simulink library "mci_models"  (R2020a)
settings: Solver=VariableStepAuto  StartTime=0.0  StopTime=10.0  RelTol=1e-3
undefined symbols (not defined in the file): x0
(part 1 of 2)
Description:
  | Library of MCI specific blocks and models.
  | 
  | Release 2023
settings Model: Creator=Andreas Mehrle  LastModifiedBy=User
settings DataIOCC: ReturnWorkspaceOutputs=off
settings DebuggingCC: ArithmeticOperatorsInVariantConditions=warning
settings SFSimCC: SimUseLocalCustomCode=off  CustomCodeUndefinedFunction=UseInterfaceOnly
settings RTWCC: RTWUseLocalCustomCode=off
settings CodeAppCC: StateflowObjectComments=on

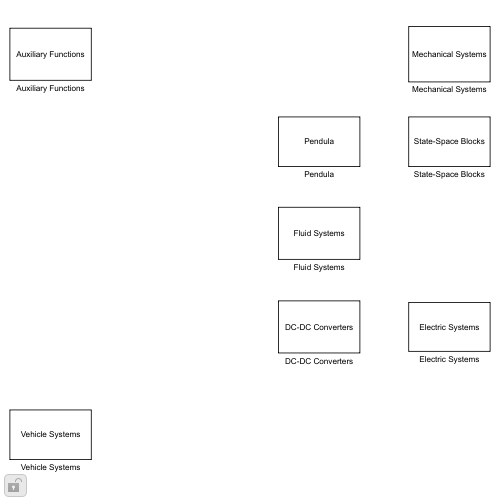
[thumbnail: Simulink's stored preview of the top-level diagram]
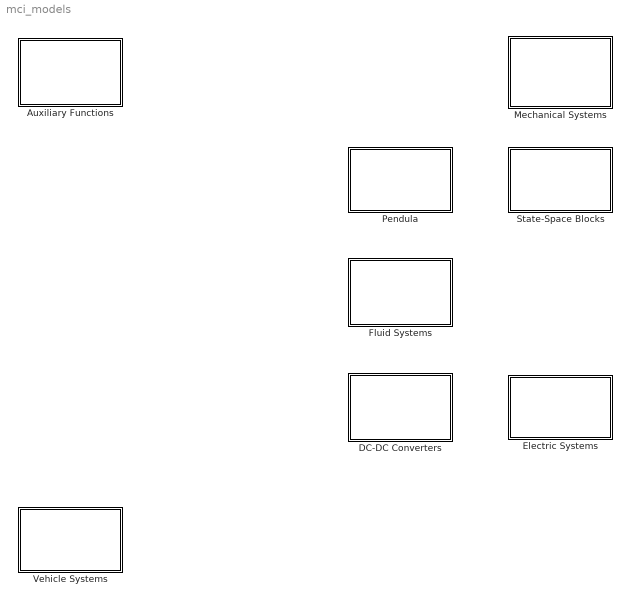
== system mci_models ==
  Auxiliary Functions : Subsystem
      mask Display: disp(get_param(gcb,'Name'))
  DC-DC Converters : Subsystem
      mask Display: disp(get_param(gcb,'Name'))
  Electric Systems : Subsystem
      mask Display: disp(get_param(gcb,'Name'))
  Fluid Systems : Subsystem
      mask Display: disp(get_param(gcb,'Name'))
  Mechanical Systems : Subsystem
      mask Display: disp(get_param(gcb,'Name'))
  Pendula : Subsystem
      mask Display: disp(get_param(gcb,'Name'))
  State-Space Blocks : Subsystem
      mask Display: disp(get_param(gcb,'Name'))
  Vehicle Systems : Subsystem
      mask Display: disp(get_param(gcb,'Name'))

== system mci_models/Auxiliary Functions ==
  Friction model : Subsystem  mask(Friction Function){c=[1 20 0.5 0]}
      mask prompts: c "Friction parameters"
      mask help:
      | Block computes non-linear friction coefficient.
      |
      | Inputs:
      |  - v ... vehicle velocity (m/s)
      |  - v_w ... wheel velocity (m/s)
      |
      | Outputs:
      |  - lambda ... slip
      |  - mu ... friction coefficient
      mask init:
      | p.c=c;
      mask DialogControl DescTextVar Prompt: Engine characteristics
      mask Display:
      | l=0:1/20:1;
      | m=c(1)*(1-exp(-c(2)*l))-c(3)*l;
      | 
      | color('white')
      | plot([-0.2 -0.2],[-0.2 1.3]);
      | plot([-0.2 1.3],[-0.2 -0.2]);
      | 
      | color('black')
      | plot(l,m)
      | plot([0 1 1 0 0],[0 0 1 1 0])
      | %plot([0 0],[0 1])
      | %text(1.1,0.09,'l')
      | %text(0.02,1.2,'mu')
      | 
      | port_label('input',1,'v')
      | port_label('input',2,'v_w','texmode','on')
      | port_label('output',1,'\lambda','texmode','on')
      | port_label('output',2,'\mu','texmode','on')
  Polynomial : Subsystem  mask(Polynomial Function){p=[-4 4 0]}
      mask prompts: p "Coefficients ([p_n p_n-1 ... p_1 p_0])"
      mask help: Establishes polynomial relation between input and output.
      mask DialogControl DescTextVar Prompt: Engine characteristics
      mask Display:
      | wmax=max(roots(p));
      | w=0:wmax/10:wmax;
      | %wmax=max(w);
      | ymax=max(polyval(p,w));
      | 
      | color('white')
      | plot([-0.2*wmax -0.2*wmax],[-0.2*ymax 1.3*ymax]);
      | plot([-0.2*wmax 1.3*wmax],[-0.2*ymax -0.2*ymax]);
      | 
      | color('black')
      | plot(w,polyval(p,w))
      | plot([0 wmax wmax 0 0],[0 0 ymax ymax 0])
      | %plot([0 0],[0 ymax])
      | %text(1.1*wmax,0.09*ymax,'u')
      | %text(0.02*wmax,1.2*ymax,'y')
      | 
      | %port_label('input',1,'u')
      | %port_label('output',1,'y')
  Trajectory : Subsystem  mask(Trajectory Generator){t1=1, dt=1, y1=0, y2=1, n=5, m=0}
      mask prompts: t1 "Start time (s)"; dt "Duration (s)"; y1 "Start value"; y2 "End value"; n "Order"; m "Derivatives"
      mask help:
      | Generates polynomial trajectory of different order with smooth beginning and end.
      |
      | Inputs: none
      |
      | Outputs:
      |  - y ... trajectory
      |  - dy ... time derivative of y (optional)
      |  - ddy ... second derivative of y (optional)
      |
      | Before start time and after ending y is kept constant and all derivatives become 0.
      mask init:
      | p.t1=t1;
      |     p.t2=t1+dt;
      |     p.dt=dt;
      |     p.y1=y1;
      |     p.y2=y2;
      | 
      |     p.n=str2num(get_param(gcb,'n'));
      |     if p.n==3
      |         p.p=[-2 3 0 0];
      |         p.dp=[-6 6 0];
      |         p.ddp=[-12 6];
      |     elseif p.n==5
      |         p.p=[6 -15 10 0 0 0];
      |         p.dp=[30 -60 30 0 0];
      |         p.ddp=[120 -180 60 0];
      |     elseif p.n==7
      |         p.p=[-20 70 -84 35 0 0 0 0];
      |         p.dp=[-140 420 -420 140 0 0 0];
      |         p.ddp=[-840 2100 -1680 420 0 0];
      |     end
      | 
      |     p.m=str2num(get_param(gcb,'m'));
      |     if p.m==0
      |         if (getSimulinkBlockHandle([gcb, '/dy']) ~= -1)             % If it DOES exist (dy)
      |                 ho = get_param([gcb, '/dy'], 'LineHandles');        % we get the line handles to eliminate them first
      |                 delete_line(ho.Inport);                             % we delete the line
      |                 delete_block([gcb, '/dy']);                    % we delete the block
      |         end
      |         if (getSimulinkBlockHandle([gcb, '/ddy']) ~= -1)             % If it DOES exist (dy)
      |                 ho = get_param([gcb, '/ddy'], 'LineHandles');        % we get the line handles to eliminate them first
      |                 delete_line(ho.Inport);                             % we delete the line
      |                 delete_block([gcb, '/ddy']);                    % we delete the block
      |         end
      |     elseif p.m==1
      |         if (getSimulinkBlockHandle([gcb, '/dy']) == -1)             % If it DOES NOT exist (dy)
      |                 add_block('simulink/Sinks/Out1',[gcb, '/dy']);% add the block
      |                 set_param([gcb, '/dy'],'position',[285    53   315    67]);    % we place it somewhere
      |                 ho = get_param([gcb, '/dy'], 'PortHandles');               % we get the port handles of the new inport port
      |                 gen = get_param([gcb, '/tragen'], 'PortHandles');           % we get the port handles of the product block
      |                 add_line(gcb,gen.Outport(2),ho.Inport(1));                       % we create the connection between new input outport and appropriate product inport
      |         end
      |         if (getSimulinkBlockHandle([gcb, '/ddy']) ~= -1)             % If it DOES exist (dy)
      |                 ho = get_param([gcb, '/ddy'], 'LineHandles');        % we get the line handles to eliminate them first
      |                 delete_line(ho.Inport);                             % we delete the line
      |                 delete_block([gcb, '/ddy']);                    % we delete the block
      |         end
      |     elseif p.m==2
      |         if (getSimulinkBlockHandle([gcb, '/dy']) == -1)             % If it DOES NOT exist (dy)
      |                 add_block('simulink/Sinks/Out1',[gcb, '/dy']);% add the block
      |                 set_param([gcb, '/dy'],'position',[285    53   315    67]);    % we place it somewhere
      |                 ho = get_param([gcb, '/dy'], 'PortHandles');               % we get the port handles of the new inport port
      |                 gen = get_param([gcb, '/tragen'], 'PortHandles');           % we get the port handles of the product block
      |                 add_line(gcb,gen.Outport(2),ho.Inport(1));                       % we create the connection between new input outport and appropriate product inport
      |         end
      |         if (getSimulinkBlockHandle([gcb, '/ddy']) == -1)             % If it DOES NOT exist (dy)
      |                 add_block('simulink/Sinks/Out1',[gcb, '/ddy']);% add the block
      |                 set_param([gcb, '/ddy'],'position',[285    88   315   102]);    % we place it somewhere
      |                 ho = get_param([gcb, '/ddy'], 'PortHandles');               % we get the port handles of the new inport port
      |                 gen = get_param([gcb, '/tragen'], 'PortHandles');           % we get the port handles of the product block
      |                 add_line(gcb,gen.Outport(3),ho.Inport(1));                       % we create the connection between new input outport and appropriate product inport
      |         end
      | 
      |     end
      mask TypeOptions n: 3 | 5 | 7
      mask TypeOptions m: 0 | 1 | 2
      mask DialogControl DescTextVar Prompt: Engine characteristics
      mask Display:
      | t=0:p.dt/10:p.dt;
      | tmax=p.t2;
      | y=p.y1+(p.y2-p.y1)*polyval(p.p,t/p.dt);
      | ymax=max(y);
      | 
      | color('white')
      | plot([-0.2*tmax -0.2*tmax],[-0.2*ymax 1.3*ymax]);
      | plot([-0.2*tmax 1.3*tmax],[-0.2*ymax -0.2*ymax]);
      | 
      | color('black')
      | plot([0 t+p.t1],[p.y1 y])
      | plot([0 tmax tmax 0 0],[0 0 ymax ymax 0])
      | %plot([0 0],[0 ymax])
      | %text(1.1*tmax,0.09*ymax,'t')
      | %text(0.02*tmax,1.2*ymax,'y')
      | text(0.1*tmax,0.8*ymax,['n=',num2str(p.n)])
      | 
      | %port_label('output',1,'y')
      | %if p.n>1
      | %    port_label('output',2,'\dot{y}','texmode','on')
      | %end

== system mci_models/DC-DC Converters ==
  Buck Converter : Subsystem  mask{L=1, R=1, C=1, G=1, ui=1, x0=[0;0]}
      mask prompts: L "L (H)"; R "R (Ohm)"; C "C (F)"; G "G (S)"; ui "Supply voltage (V)"; x0 "Initial state [i_L;u_C]"
      mask DialogControl DescTextVar Prompt: Cuk Converter
      mask Display:
      | % labels
      | %port_label('input',1,'u_i','texmode','on')
      | %port_label('input',2,'d')
      | %port_label('output',1,'x')
      | % circuit
      | plot([0.15 0.30],[0.7 0.7])
      | plot([0.29 0.4 0.85 0.85],[0.6 0.7 0.7 0.6])
      | %patch([0.15 0.3 0.3 0.15 0.15],[0.73 0.73 0.62 0.62 0.73],[0 0 0])
      | %plot([0.39 0.39],[0.8 0.6])
      | %plot([0.415 0.415],[0.8 0.6])
      | patch([0.47 0.62 0.62 0.47 0.47],[0.73 0.73 0.62 0.62 0.73],[0 0 0])
      | %plot([0.35 0.35 0.4],[0.7 0.5 0.5])
      | %plot([0.45 0.45],[0.7 0.5])
      | plot([0.3 0.3],[0.62 0.2])
      | plot([0.7 0.7],[0.7 0.47])
      | plot([0.65 0.75],[0.47 0.47])
      | plot([0.65 0.75],[0.43 0.43])
      | plot([0.7 0.7],[0.43 0.2])
      | plot([0.815 0.875 0.875 0.815 0.815],[0.6 0.6 0.3 0.3 0.6])
      | plot([0.15 0.85 0.85],[0.2 0.2 0.3])
  Cuk Converter : Subsystem  mask{L1=1, R1=1, C1=1, L2=1, R2=1, C2=1, G=1, ui=1, x0_copy=[0;0;1e-6;0]}
      mask prompts: L1 "L1 (H)"; R1 "R1 (Ohm)"; C1 "C1 (F)"; L2 "L2 (H)"; R2 "R2 (Ohm)"; C2 "C2 (F)"; G "G (S)"; ui "Supply voltage"; x0_copy "Initial state [i1;i2;uc1;uc2]"
      mask init:
      | p.L1=L1;
      | p.R1=R1;
      | p.C1=C1;
      | p.L2=L2;
      | p.R2=R2;
      | p.C2=C2;
      | p.G=G;
      | p.ui=ui;
      mask DialogControl DescTextVar Prompt: Cuk Converter
      mask Display:
      | % labels
      | %port_label('input',1,'u_i','texmode','on')
      | %port_label('input',2,'d')
      | %port_label('output',1,'x')
      | % circuit
      | plot([0.05 0.39],[0.7 0.7])
      | plot([0.415 0.9 0.9],[0.7 0.7 0.6])
      | patch([0.15 0.3 0.3 0.15 0.15],[0.73 0.73 0.62 0.62 0.73],[0 0 0])
      | plot([0.39 0.39],[0.8 0.6])
      | plot([0.415 0.415],[0.8 0.6])
      | patch([0.5 0.65 0.65 0.5 0.5],[0.73 0.73 0.62 0.62 0.73],[0 0 0])
      | plot([0.35 0.35 0.4],[0.7 0.5 0.5])
      | plot([0.45 0.45],[0.7 0.5])
      | plot([0.38 0.45 0.45],[0.53 0.35 0.2])
      | plot([0.75 0.75],[0.7 0.47])
      | plot([0.7 0.8],[0.47 0.47])
      | plot([0.7 0.8],[0.43 0.43])
      | plot([0.75 0.75],[0.43 0.2])
      | plot([0.865 0.925 0.925 0.865 0.865],[0.6 0.6 0.3 0.3 0.6])
      | plot([0.1 0.9 0.9],[0.2 0.2 0.3])
  RL-Load : Subsystem  mask{L=1, R=1, ui=1, x0=0}
      mask prompts: L "L (H)"; R "R (Ohm)"; ui "Supply voltage (V)"; x0 "Initial state [i_L]"
      mask DialogControl DescTextVar Prompt: Cuk Converter
      mask Display:
      | % labels
      | %port_label('input',1,'u_i','texmode','on')
      | %port_label('input',1,'d')
      | %port_label('output',1,'x')
      | % circuit
      | plot([0.15 0.50 0.5 0.55],[0.9 0.9 0.8 0.7])
      | plot([0.3 0.3 0.35],[0.9 0.8 0.7])
      | plot([0.3 0.3 0.35],[0.7 0.3 0.2])
      | plot([0.3 0.3],[0.2 0.1])
      | plot([0.5 0.5 0.55],[0.7 0.3 0.2])
      | plot([0.5 0.8 0.8 0.3],[0.6 0.6 0.4 0.4])
      | patch([0.65 0.75 0.75 0.65],[0.375 0.375 0.425 0.425],[0 0 0])
      | %plot([0.3 0.3],[0.62 0.2])
      | %plot([0.7 0.7],[0.7 0.47])
      | %plot([0.65 0.75],[0.47 0.47])
      | %plot([0.65 0.75],[0.43 0.43])
      | %plot([0.7 0.7],[0.43 0.2])
      | %plot([0.815 0.875 0.875 0.815 0.815],[0.6 0.6 0.3 0.3 0.6])
      | plot([0.15 0.5 0.5],[0.1 0.1 0.2])

== system mci_models/Electric Systems ==
  GPS-IMU Sensor : Subsystem  mask{T=1, D=1, var_IMU=0.1, a0=0.1}
      mask prompts: T "Sampling time (s)"; D "Quantization (m)"; var_IMU "Noise variation (m^2/s^4)"; a0 "Offset (m/s^2)"
      mask DialogControl Container3 Prompt: GPS
      mask DialogControl Container4 Prompt: IMU
      mask Display:
      | image(imread('grafics/gyro.png'))
      | 
      | % labels
      | port_label('input',1,'u')
      | port_label('output',1,'y_{GPS}','texmode','on')
      | port_label('output',2,'a_{IMU}','texmode','on')
  Magnetic Levitation : Subsystem  mask{y0=1, m=1, R=1, L0=1, L1=1, g=9.81, x0=[0;0;0]}
      mask prompts: y0 "Operating distance (m)"; m "Levitated mass (kg)"; R "Coil resistance (Ohm)"; L0 "Coil inductance (H)"; L1 "Sphere inductance (H)"; g "Gravitational acceleration (m/s^2)"; x0 "Initial state [y;v;i]"
      mask init:
      | p.y0=y0;
      | p.m=m;
      | p.R=R;
      | p.L0=L0;
      | p.L1=L1;
      | p.g=g;
      mask Display:
      | patch([0.580 0.576 0.565 0.547 0.525 0.500 0.475 0.453 0.435 0.424 0.420 0.424 0.435 0.453 0.475 0.500 0.525 0.547 0.565 0.576 0.580 ],[0.500 0.533 0.563 0.586 0.601 0.607 0.601 0.586 0.563 0.533 0.500 0.467 0.437 0.414 0.399 0.393 0.399 0.414 0.437 0.467 0.500 ])
      | patch([0.4 0.6 0.6 0.4],[0.95 0.95 0.85 0.85],[0.5 0.5 0.5])
      | plot([0.177 0.250 0.330 0.414 0.500 0.586 0.670 0.750 0.823 ],[0.407 0.347 0.303 0.276 0.267 0.276 0.303 0.347 0.407 ])
      | plot([0.235 0.296 0.361 0.430 0.500 0.570 0.639 0.704 0.765 ],[0.515 0.465 0.429 0.407 0.400 0.407 0.429 0.465 0.515 ])
      | plot([0.294 0.341 0.392 0.445 0.500 0.555 0.608 0.659 0.706 ],[0.622 0.584 0.556 0.539 0.533 0.539 0.556 0.584 0.622 ])
      | plot([0.353 0.387 0.423 0.461 0.500 0.539 0.577 0.613 0.647 ],[0.730 0.703 0.683 0.671 0.667 0.671 0.683 0.703 0.730 ])
      | plot([0.7 0.1 0.1 0.6],[0 0 1 1])
      | % labels
      | port_label('input',1,'u')
      | port_label('output',1,'x')

== system mci_models/Fluid Systems ==
  Bioreactor : Subsystem  mask{cg0=0, mu0=0, k0=0, k1=0, k2=0, alpha=0, x0=[0;0]}
      mask prompts: cg0 "Inflow concentration glucose (kg/m^3)"; mu0 "Growth rate (1/[t])"; k0 "Affinity constant (kg/m^3)"; k1 "Linear affinity constant"; k2 "Quadratic affinity constant (m^3/kg)"; alpha "Yield rate"; x0 "Initial state [c_c;c_g]"
      mask init:
      | p.cg0=cg0;
      | p.mu0=mu0;
      | p.k0=k0;
      | p.k1=k1;
      | p.k2=k2;
      | p.alpha=alpha;
      mask Display:
      | image(imread('grafics/bioreactor.png'))
      | 
      | port_label('input',1,'q')
      | port_label('output',1,'c')
  Fan Model : Subsystem  mask{K1=1, tau1=1, K2=1, tau2=1, w_on=1, w_off=1, sensorType=off, T=1}
      mask prompts: K1 "Gain (rad/s V)"; tau1 "Time constant (s)"; K2 "Gain (rad/s V)"; tau2 "Time constant (s)"; w_on "Breakoff speed (rad/s)"; w_off "Freeze speed (rad/s)"; sensorType "Enable discrete sensing"; T "Sampling time for discrete sensing (s)"
      mask init:
      | p.T=T;
      | maskHandle=Simulink.Mask.get(gcb);
      | if sensorType==1
      |     set_param([gcb,'/Sensor1'],'Commented','off');
      |     set_param([gcb,'/Sensor2'],'Commented','off');
      |     maskHandle.Parameters(1,8).Enabled='on';
      | else
      |     set_param([gcb,'/Sensor1'],'Commented','through');
      |     set_param([gcb,'/Sensor2'],'Commented','through');
      |     maskHandle.Parameters(1,8).Enabled='off';
      | end
      mask DialogControl DescTextVar Prompt: BB8 model
      mask DialogControl Fan1 Prompt: Fan 1
      mask DialogControl Fan2 Prompt: Fan 2
      mask DialogControl Container5 Prompt: Sensor
      mask Display:
      | image(imread('grafics/turbine.png'))
      | 
      | port_label('input',1,'u')
      | port_label('output',1,'w1')
      | port_label('output',2,'w2')
  Pneumatic Cylinder : Subsystem  mask{m=1, A=1, k=1, b=0.1, x0=[1;0]}
      mask prompts: m "Piston mass (kg)"; A "Piston area (m^2)"; k "Spring konstant (N/m)"; b "Friction constant (N s/m)"; x0 "Initial state [x;v] (p will be chosen to match the spring force)"
      mask init:
      | p.m=m;
      | p.A=A;
      | p.k=k;
      | p.b=b;
      | x0(3)=x0(1)*p.k/p.A;
      mask DialogControl DescTextVar Prompt: Nonlinear pneumatic cylinder with ideal gas properties.
      mask Display:
      | % bar
      | plot([0.35,0.9],[0.5,0.5])
      | % piston
      | %plot([0.4,0.4,0.35,0.35,0.4],[0.3,0.7,0.7,0.3,0.3])
      | patch([0.42,0.42,0.38,0.38,0.42],[0.3,0.66,0.66,0.3,0.3],[0.5,0.5,0.5])
      | % case
      | plot([0.65,0.65,0.1,0.1,0.65,0.65],[0.475,0.3,0.3,0.7,0.7,0.525])
      | % spring
      | plot([0.4,0.45,0.5,0.55,0.6,0.65],[0.3,0.7,0.3,0.7,0.3,0.7])
      | % labels
      | port_label('input',1,'q')
      | port_label('output',1,'x')
  Tank with Outflow : Subsystem  mask{At=1, Ao=0.1, rho=1, zeta=0, g=9.81, h0=1}
      mask prompts: At "Tank section (m^2)"; Ao "Outflow section (m^2)"; rho "Fluid density (kg/m^3)"; zeta "Friction loss coefficient"; g "Gravitational acceleration (m/s^2)"; h0 "Initial height (m)"
      mask init:
      | p.At=At;
      | p.Ao=Ao;
      | p.rho=rho;
      | p.zeta=zeta;
      | p.g=g;
      mask DialogControl DescTextVar Prompt: Nonlinear tank with outflow
      mask Display:
      | patch([0.35 0.35 0.3 0.3],[0.75 0.6 0.6 0.75],[0.5 0.5 0.5])
      | patch([0.25 0.75 0.75 0.25],[0.6 0.6 0.2 0.2],[0.5 0.5 0.5])
      | patch([0.47 0.53 0.53 0.47],[0.2 0.2 0.05 0.05],[0.5 0.5 0.5])
      | plot([0.1 0.34 0.34 0.27 0.27 0.1],[1 1 0.8 0.8 0.88 0.88])
      | plot([0.22 0.22 0.44 0.44],[0.7 0.18 0.18 0.12])
      | plot([0.76 0.76 0.53 0.53],[0.7 0.18 0.18 0.12])
      | 
      | port_label('input',1,'qi')
      | port_label('output',1,'h')
      | port_label('output',2,'qo')

== system mci_models/Mechanical Systems ==
  Elevator : Subsystem  mask{m=1, J=1, r=1, g=9.81, b1=1, b2=0.1, k=1e3, x0=[0;1;0;0], display=off}
      mask prompts: m "Mass cabin (kg)"; J "Moment of inertia engine (kg m^2)"; r "Wheel radius (m)"; g "Gravitational acceleration (m/s^2)"; b1 "Translational friction (N s/m)"; b2 "Rotational friction (N m s)"; k "Rope stiffness (N)"; x0 "Initial state [x;phi;v;w]"; display "Activate real-time visualization"
      mask init:
      | p.r=r;
      | p.m=m;
      | p.J=J;
      | p.g=g;
      | p.b1=b1;
      | p.b2=b2;
      | p.k=k;
      | %x0(2)=x0(1)/(r*(m*g/k+1));
      settings: MinAlgLoopOccurrences=on
      mask DialogControl DescTextVar Prompt: Nonlinear pendulum on cart model
      mask Display:
      | plot([0,1],[0.05,0.05])
      | plot([0.4,0.4,0.6,0.6,0.4],[0.2,0.5,0.5,0.2,0.2])
      | plot([0.5,0.5],[0.5,1])
      | % labels
      | port_label('input',1,'M')
      | port_label('output',1,'x')
      | port_label('output',2,'e')
  Lunar Lander : Subsystem  mask{vt=0, g=9.81, x0=[1;0;1]}
      mask prompts: vt "Thruster exit velocity (m/s)"; g "Gravitational acceleration (m/s^2)"; x0 "Initial state [h,v,m]"
      mask init:
      | p.vt=vt;
      | p.g=g;
      mask DialogControl DescTextVar Prompt: Lunar Lander Model
      mask Display:
      | image(imread('grafics/lander.png'))
      | 
      | port_label('input',1,'q')
      | port_label('output',1,'x')
  Segway Model : Subsystem  mask{m0=1, m1=1, I0=0, I1=0, r=1, s=1, b0=1, b1=0, g=9.81, x0=[0;0;0;0], display=on}
      mask prompts: m0 "Wheel mass (kg)"; m1 "Pendulum mass (kg)"; I0 "Wheel moment of inertia (kg m^2)"; I1 "Pendulum moment of inertia (kg m^2)"; r "Wheel radius"; s "Distance of pendulum COG from hub (m)"; b0 "Rolling friction coefficient wheel (N m s/rad)"; b1 "Turning friction coefficient hub (N m s/rad)"; g "Gravitational acceleration (m/s^2)"; x0 "Initial state [a;w;da;dw]"; display "Activate real-time visualization"
      mask init:
      | p.m0=m0;
      | p.m1=m1;
      | p.I0=(m0+m1)*r^2+I0;
      | p.I1=m1*s^2+I1;
      | p.I01=m1*r*s;
      | p.b1=b1;
      | if b1==0;
      |     p.nu=b0/1e-6;
      | else
      |     p.nu=b0/b1;
      | end
      | p.g=g/r;
      mask DialogControl DescTextVar Prompt: BB8 model
      mask Display:
      | image(imread('grafics/segway.png'))
      | 
      | port_label('input',1,'M')
      | port_label('output',1,'x')

== system mci_models/Pendula ==
  Double Pendulum on Cart : Subsystem  mask{s1=1, s2=1, l1=1, m0=1, m1=1, m2=1, I1=0, I2=0, g=9.81, b0=0.1, b1=0.1, b2=0.1, x0=[0;0;0;0;0;0], display=off}
      mask prompts: s1 "Distance of pendulum 1 COG from hinge point (m)"; s2 "Distance of pendulum 2 COG from hinge point (m)"; l1 "Length of pendulum 1 (m)"; m0 "Mass cart (kg)"; m1 "Mass pendulum 1 (kg)"; m2 "Mass pendulum 2 (kg)"; I1 "Moment of inertia pendulum 1 (kg m^2)"; I2 "Moment of inertia pendulum 2 (kg m^2)"; g "Gravitational acceleration (m/s^2)"; b0 "Translational friction (N s/m)"; b1 "Rotational friction joint 1 (N m s)"; b2 "Rotational friction joint 2 (N m s)"; x0 "Initial state [x;phi1;phi2;v;w1;w2]"; display "Activate real-time visualization"
      mask init:
      | p.M=m0+m1+m2;
      | p.I11=I1+m1*s1^2+m2*l1^2;
      | p.I22=I2+m2*s2^2;
      | p.I12=m2*l1*s2;
      | p.I2p=m2*s2;
      | p.I12p=m1*s1+m2*l1;
      | p.g=g;
      | p.b0=b0;
      | p.b1=b1;
      | p.b2=b2;
      mask Display:
      | plot([0,1],[0.05,0.05])
      | plot([0.3,0.3,0.7,0.7,0.3],[0.1,0.4,0.4,0.1,0.1])
      | plot([0.5,0.6,0.4],[0.25,0.65,1])
      | % labels
      | port_label('input',1,'F')
      | port_label('output',1,'x')
  Mathematical Pendulum : Subsystem  mask{m=1, l=1, k=0, b=0.1, g=9.81, x0=[0;0], display=off}
      mask prompts: m "Mass (kg)"; l "Pendulum length (m)"; k "Spring constant (N m/rad)"; b "Friction coefficient (N m s/rad)"; g "Gravitational acceleration (m/s^2)"; x0 "Initial state [phi;w]"; display "Activate real-time visualization"
      mask init:
      | p.m=m;
      | p.l=l;
      | p.k=k;
      | p.b=b;
      | p.g=g;
      mask DialogControl DescTextVar Prompt: Nonlinear mathematical pendulum
      mask Display:
      | % support
      | plot([0.3 0.7],[1 1])
      | plot([0.45 0.5 0.55],[1 0.9 1])
      | % pendulum
      | plot([0.5 0.33],[0.9 0.22])
      | text(0.3,0.2,'O')
      | % labels
      | port_label('input',1,'M')
      | port_label('output',1,'x')
  Motion Controlled Double Pendulum : Subsystem  mask{g=9.81, x0=[0;0;0;0;0], display=off, l1=1, m2=1, m1=1, s2=1, s1=1, I2=0, b2=0.1, I1=0, b1=0.1}
      mask prompts: g "Gravitational acceleration (m/s^2)"; x0 "Initial state [x;phi1;phi2;w1;w2]"; display "Activate real-time visualization"; l1 "Length (m)"; m2 "Mass (kg)"; m1 "Mass (kg)"; s2 "Distance of COG from hinge point (m)"; s1 "Distance of COG from hinge point (m)"; I2 "Moment of inertia (kg m^2)"; b2 "Rotational friction (N m s)"; I1 "Moment of inertia (kg m^2)"; b1 "Rotational friction (N m s)"
      mask init:
      | p.I11=I1+m1*s1^2+m2*l1^2;
      | p.I22=I2+m2*s2^2;
      | p.I12=m2*l1*s2;
      | p.I2p=m2*s2;
      | p.I12p=m1*s1+m2*l1;
      | p.g=g;
      | p.b1=b1;
      | p.b2=b2;
      mask DialogControl Container3 Prompt: Pendulum 1
      mask DialogControl Container4 Prompt: Pendulum 2
      mask Display:
      | % ground
      | plot([0,1],[0.05,0.05])
      | % cart
      | plot([0.3,0.3,0.7,0.7,0.3],[0.1,0.3,0.3,0.1,0.1])
      | % pendulum
      | plot([0.5,0.6,0.4],[0.3,0.63,0.95])
      | % motion control
      | plot([0,0.3],[0.2,0.2])
      | plot([0.25,0.3,0.25],[0.15,0.2,0.25])
      | % labels
      | port_label('input',1,'v')
      | port_label('output',1,'x')
      | 
      | 
      | %plot([0,1],[0.05,0.05])
      | %plot([0.3,0.3,0.7,0.7,0.3],[0.1,0.4,0.4,0.1,0.1])
      | %plot([0.5,0.6,0.4],[0.25,0.65,1])
      | %plot([0,0.3],[0.25,0.25])
      | %plot([0.25,0.3,0.25],[0.2,0.25,0.3])
  Motion Controlled Pendulum : Subsystem  mask{s=1, m1=1, J=0, g=9.81, b1=0.1, x0=[0;0;0;0], display=off}
      mask prompts: s "Distance of pendulum COG from hinge point (m)"; m1 "Mass pendulum (kg)"; J "Moment of inertia pendulum"; g "Gravitational acceleration (m/s^2)"; b1 "Rotational friction (N m s)"; x0 "Initial state [x;phi;w]"; display "Activate real-time visualization"
      mask init:
      | p.s=s;
      | p.m1=m1;
      | p.J1=J;
      | p.g=g;
      | p.b1=b1;
      settings: MinAlgLoopOccurrences=on
      mask DialogControl DescTextVar Prompt: Nonlinear pendulum on cart model
      mask Display:
      | % ground
      | plot([0,1],[0.05,0.05])
      | % cart
      | plot([0.3,0.3,0.7,0.7,0.3],[0.1,0.3,0.3,0.1,0.1])
      | % pendulum
      | plot([0.5,0.6],[0.3,0.95])
      | % motion control
      | plot([0,0.3],[0.2,0.2])
      | plot([0.25,0.3,0.25],[0.15,0.2,0.25])
      | % labels
      | port_label('input',1,'v')
      | port_label('output',1,'x')
  Pendulum on Cart : Subsystem  Description=|  mask{s=1, m0=1, m1=1, J=0, g=9.81, b0=0, b1=0.1, x0=[0;0;0;0], display=off}
      | Simple model for pendulum on force driven slider. The states are x=[y v] where y is the
      | (horizontal) position and v the velocity of the slider. As input a force is taken u=F.
      | 
      | For the slider only its mass and the friction koefficient with the surface needs to be provided.
      | For the pendulum parameters include mass, distance of COG from hinge point, moment of
      | inertia around the COG for the pendulum and the friction coefficient of the rotatory motion.
      mask prompts: s "Distance of pendulum COG from hinge point (m)"; m0 "Mass cart (kg)"; m1 "Mass pendulum (kg)"; J "Moment of inertia pendulum"; g "Gravitational acceleration (m/s^2)"; b0 "Translational friction (N s/m)"; b1 "Rotational friction (N m s)"; x0 "Initial state [y;phi;v;w]"; display "Activate real-time visualization"
      mask init:
      | p.s=s;
      | p.m0=m0
      | p.m1=m1;
      | p.J=J;
      | p.g=g;
      | p.b0=b0;
      | p.b1=b1;
      settings: MinAlgLoopOccurrences=on
      mask DialogControl DescTextVar Prompt: Nonlinear pendulum on cart model
      mask Display:
      | plot([0,1],[0.05,0.05])
      | plot([0.3,0.3,0.7,0.7,0.3],[0.1,0.4,0.4,0.1,0.1])
      | plot([0.5,0.6],[0.25,1])
      | % labels
      | port_label('input',1,'F')
      | port_label('output',1,'x')

== system mci_models/State-Space Blocks ==
  Continuous State-Space : Subsystem  mask{A=1, B=1, C=1, D=1, x0=0}
      mask prompts: x0 "Initial conditions:"
      mask DialogControl DescTextVar Prompt: State-space model
      mask Display:
      | % annotation
      | text(0.5,0.6,'x''=Ax+Bu','horizontalAlignment','center')
      | text(0.5,0.4,'y=Cx+Du','horizontalAlignment','center')
      | % ports
      | port_label('input',1,'u')
      | port_label('output',1,'y')
      | port_label('output',2,'x')
  Discrete State-Space : Subsystem  mask{A=1, B=1, C=1, D=1, x0=0, T=1}
      mask prompts: x0 "Initial conditions:"; T "Sampling time"
      mask DialogControl DescTextVar Prompt: State-space model
      mask Display:
      | % annotation
      | text(0.5,0.6,texlabel('x_{k+1}=Ax_k+Bu_k'),'horizontalAlignment','center','Interpreter','tex')
      | text(0.5,0.4,'y_k=Cx_k+Du_k','horizontalAlignment','center','Interpreter','tex')
      | % ports
      | port_label('input',1,'u_k','Interpreter','tex')
      | port_label('output',1,'y_k','Interpreter','tex')
      | port_label('output',2,'x_k','Interpreter','tex')

== system mci_models/Vehicle Systems ==
  Car Dynamics : Subsystem  mask(Car Dynamics Model){m=1, cf=1, cd=1, rho=1.25, A=1, g=9.81, x0=0}
      mask prompts: m "Car mass (kg)"; cf "Friction coefficient"; cd "Drag coefficient"; rho "Air density (kg/m^3)"; A "Projected section area (m^2)"; g "Gravitational acceleration (m/s^2)"; x0 "Initial velocity [v0]"
      mask help:
      | Calculates the one-dimensional dynamics of a vehicle.
      |
      | Inputs:
      |  - phi ... road inclination (rad)
      |  - F ... thrust force (N)
      |
      | Outputs:
      |  - a ... acceleration (m/s^2)
      |  - v ... velocity (m/s)
      |
      | Mechanical (velocity proportional) and aerodynamic drag are considered by the respective coefficients.
      mask init:
      | p.m=m;
      | p.cd=cd;
      | p.cf=cf;
      | p.rho=rho;
      | p.A=A;
      | p.g=g;
      mask DialogControl DescTextVar Prompt: Car dynamics
      mask Display:
      | image(imread('grafics/car1.png'))
      | 
      | port_label('input',1,'\phi','texmode','on')
      | port_label('input',2,'F')
      | port_label('output',1,'a')
      | port_label('output',2,'v')
  Car Kinematics : Subsystem  mask(Car Kinematics Model){l=1, phimax=1, x0=[0;0;0]}
      mask prompts: l "Wheelbase (m)"; phimax "Maximum steering angle (rad)"; x0 "Initial state [x;y;phi]"
      mask help:
      | Computes two-dimensional (in-plane) kinematics of a vehicle.
      |
      | Inputs:
      |  - v ... translational velocity (m/s)
      |  - alpha ... steering angle (rad)
      |
      | Outputs:
      |  - x ... state [x-position, y-position, heading angle]
      |  - dx ... derivative of x [x-velocity, y-velocity, angular rotation rate]
      |
      | Steering angle can be limited to a maximum value.
      mask DialogControl DescTextVar Prompt: Kinematic model of a car
      mask Display:
      | image(imread('grafics/car2.png'))
      | 
      | port_label('input',1,'v')
      | port_label('input',2,'\alpha','texmode','on')
      | port_label('output',1,'x')
      | port_label('output',2,'dx')
      | % draw car
      | %patch([0.2 0.3 0.3 0.2],[0.73 0.73 0.7 0.7],[0 0 0])
      | %patch([0.7 0.8 0.8 0.7],[0.73 0.73 0.7 0.7],[0 0 0])
      | %plot([0.1 0.9 0.9 0.1 0.1],[0.7 0.7 0.3 0.3 0.7])
  Wheel Dynamics : Subsystem  mask(Wheel Dynamics Model){J=1, r=1, w0=0}
      mask prompts: J "Wheel moment of inertia (kg m^2)"; r "Radius (m)"; w0 "Initial velocity [w0]"
      mask help:
      | Computes wheel velocity from applied torque and road friction force. Usually used together with friction model.
      |
      | Inputs:
      |  - M ... engine torque (Nm)
      |  - F ... road friction force (N)
      |
      | Output:
      |  - v_w ... wheel velocity (m/s)
      |
      | Takes into account wheel dynamics by its moment of inertia.
      mask init:
      | p.J=J;
      | p.r=r;
      mask DialogControl DescTextVar Prompt: Car dynamics
      mask Display:
      | image(imread('grafics/wheel.png'))
      | 
      | port_label('input',1,'M')
      | port_label('input',2,'F')
      | port_label('output',1,'v_w','texmode','on')

== system mci_models/Auxiliary Functions/Friction model ==
  v : Inport
  w : Inport  Port=2
  MATLAB Function : MATLAB Function  TreatAsAtomicUnit=on
  l : Outport  VectorParamsAs1DForOutWhenUnconnected=off
  mu : Outport  Port=2  VectorParamsAs1DForOutWhenUnconnected=off
  wires:
  v/1 -> MATLAB Function/1(v)
  w/1 -> MATLAB Function/2(w)
  MATLAB Function/2(m) -> mu/1
  MATLAB Function/1(l) -> l/1

== system mci_models/Auxiliary Functions/Polynomial ==
  u : Inport
  MATLAB Function1 : MATLAB Function  TreatAsAtomicUnit=on
  y : Outport  VectorParamsAs1DForOutWhenUnconnected=off
  wires:
  MATLAB Function1/1(y) -> y/1
  u/1 -> MATLAB Function1/1(u)

== system mci_models/Auxiliary Functions/Trajectory ==
  Clock : Clock
  tragen : MATLAB Function  TreatAsAtomicUnit=on
  y : Outport  VectorParamsAs1DForOutWhenUnconnected=off
  wires:
  Clock/1 -> tragen/1(t)
  tragen/1(y) -> y/1

== system mci_models/DC-DC Converters/Buck Converter ==
  d : Inport
  Gain : Gain  Gain=[ui/L;0]  Multiplication=Matrix(K*u)
  Gain1 : Gain  Gain=[-R/L -1/L;1/C -G/C]  Multiplication=Matrix(K*u)
  Integrator : Integrator  InitialCondition=x0
  Sum : Sum  Inputs=|++
  x : Outport  VectorParamsAs1DForOutWhenUnconnected=off
  wires:
  Integrator/1 -> Gain1/1, x/1
  d/1 -> Gain/1
  Gain/1 -> Sum/1
  Sum/1 -> Integrator/1
  Gain1/1 -> Sum/2

== system mci_models/DC-DC Converters/Cuk Converter ==
  d : Inport
  Cuk converter1 : MATLAB Function  TreatAsAtomicUnit=on
  Integrator : Integrator  InitialCondition=x0
  x : Outport  VectorParamsAs1DForOutWhenUnconnected=off
  wires:
  d/1 -> Cuk converter1/1(d)
  Cuk converter1/1(dx) -> Integrator/1
  Integrator/1 -> x/1, Cuk converter1/2(x)

== system mci_models/DC-DC Converters/RL-Load ==
  d : Inport
  Gain : Gain  Gain=ui/L
  Gain1 : Gain  Gain=-R/L
  Integrator : Integrator  InitialCondition=x0
  Sum : Sum  Inputs=|++
  u : Outport  VectorParamsAs1DForOutWhenUnconnected=off
  wires:
  d/1 -> Gain/1
  Gain/1 -> Sum/1
  Sum/1 -> Integrator/1
  Integrator/1 -> Gain1/1, u/1
  Gain1/1 -> Sum/2

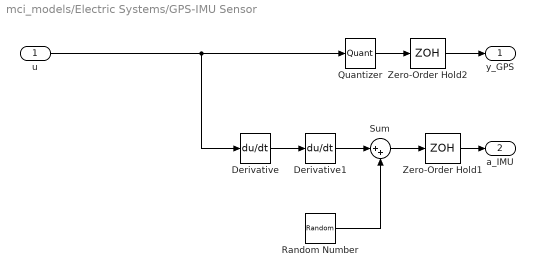
== system mci_models/Electric Systems/GPS-IMU Sensor ==
  u : Inport
  Derivative : Derivative
  Derivative1 : Derivative
  Quantizer : Quantizer  QuantizationInterval=D
  Random Number : RandomNumber  Mean=a0  Variance=var_IMU  Seed=rand()  SampleTime=T
  Sum : Sum  Inputs=|++
  Zero-Order Hold1 : ZeroOrderHold  SampleTime=T
  Zero-Order Hold2 : ZeroOrderHold  SampleTime=T
  y_GPS : Outport  VectorParamsAs1DForOutWhenUnconnected=off
  a_IMU : Outport  Port=2  VectorParamsAs1DForOutWhenUnconnected=off
  wires:
  Derivative/1 -> Derivative1/1
  Derivative1/1 -> Sum/1
  Random Number/1 -> Sum/2
  u/1 -> Derivative/1, Quantizer/1
  Quantizer/1 -> Zero-Order Hold2/1
  Zero-Order Hold2/1 -> y_GPS/1
  Zero-Order Hold1/1 -> a_IMU/1
  Sum/1 -> Zero-Order Hold1/1

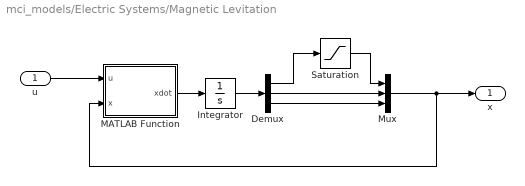
== system mci_models/Electric Systems/Magnetic Levitation ==
  u : Inport
  Demux : Demux  Outputs=3
  Integrator : Integrator  InitialCondition=x0
  MATLAB Function : MATLAB Function  TreatAsAtomicUnit=on
  Mux : Mux  Inputs=3
  Saturation : Saturate  UpperLimit=2*p.y0  LowerLimit=0
  x : Outport  VectorParamsAs1DForOutWhenUnconnected=off
  wires:
  u/1 -> MATLAB Function/1(u)
  MATLAB Function/1(xdot) -> Integrator/1
  Integrator/1 -> Demux/1
  Demux/1 -> Saturation/1
  Saturation/1 -> Mux/1
  Mux/1 -> MATLAB Function/2(x), x/1
  Demux/2 -> Mux/2
  Demux/3 -> Mux/3

== system mci_models/Fluid Systems/Bioreactor ==
  u : Inport
  Integrator : Integrator  InitialCondition=x0
  MATLAB Function : MATLAB Function  TreatAsAtomicUnit=on
  x : Outport  VectorParamsAs1DForOutWhenUnconnected=off
  wires:
  Integrator/1 -> MATLAB Function/2(x), x/1
  u/1 -> MATLAB Function/1(u)
  MATLAB Function/1(xdot) -> Integrator/1

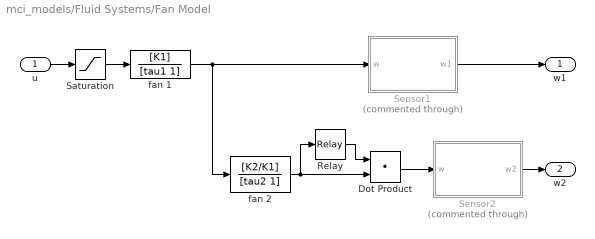
== system mci_models/Fluid Systems/Fan Model ==
  u : Inport
  Dot Product : DotProduct  InputSameDT=on  OutDataTypeStr=Inherit: Inherit via internal rule
  Relay : Relay  OnSwitchValue=w_on  OffSwitchValue=w_off
  Saturation : Saturate  UpperLimit=inf  LowerLimit=0
  Sensor1 : Subsystem  Commented=through
  Sensor2 : Subsystem  Commented=through
  fan 1 : TransferFcn  Numerator=[K1]  Denominator=[tau1 1]
  fan 2 : TransferFcn  Numerator=[K2/K1]  Denominator=[tau2 1]
  w1 : Outport  VectorParamsAs1DForOutWhenUnconnected=off
  w2 : Outport  Port=2  VectorParamsAs1DForOutWhenUnconnected=off
  wires:
  fan 1/1 -> fan 2/1, Sensor1/1(w)
  fan 2/1 -> Dot Product/2, Relay/1
  Relay/1 -> Dot Product/1
  Sensor1/1(w1) -> w1/1
  Dot Product/1 -> Sensor2/1(w)
  Sensor2/1(w2) -> w2/1
  Saturation/1 -> fan 1/1
  u/1 -> Saturation/1

== system mci_models/Fluid Systems/Pneumatic Cylinder ==
  p : Inport
  Integrator : Integrator  InitialCondition=x0
  MATLAB Function : MATLAB Function  TreatAsAtomicUnit=on
  x : Outport  VectorParamsAs1DForOutWhenUnconnected=off
  wires:
  Integrator/1 -> x/1, MATLAB Function/2(x)
  MATLAB Function/1(dx) -> Integrator/1
  p/1 -> MATLAB Function/1(u)

== system mci_models/Fluid Systems/Tank with Outflow ==
  q : Inport
  Integrator : Integrator  InitialCondition=h0
  MATLAB Function : MATLAB Function  TreatAsAtomicUnit=on
  h : Outport  VectorParamsAs1DForOutWhenUnconnected=off
  qo : Outport  Port=2  VectorParamsAs1DForOutWhenUnconnected=off
  wires:
  MATLAB Function/1(qo) -> qo/1
  MATLAB Function/2(hdot) -> Integrator/1
  Integrator/1 -> MATLAB Function/2(h), h/1
  q/1 -> MATLAB Function/1(qi)

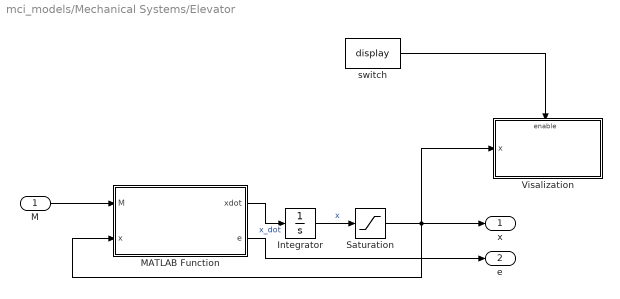
== system mci_models/Mechanical Systems/Elevator ==
  M : Inport
  Integrator : Integrator  InitialCondition=x0
  MATLAB Function : MATLAB Function  TreatAsAtomicUnit=on
  Saturation : Saturate  UpperLimit=[inf;inf;inf;inf]  LowerLimit=[-inf;1;-inf;-inf]
  Visalization : Subsystem  TreatAsAtomicUnit=on
  switch : Constant  Value=display
  x : Outport  VectorParamsAs1DForOutWhenUnconnected=off
  e : Outport  Port=2  VectorParamsAs1DForOutWhenUnconnected=off
  wires:
  M/1 -> MATLAB Function/1(M)
  Integrator/1 -> Saturation/1  "x"
  MATLAB Function/1(xdot) -> Integrator/1  "x_dot"
  switch/1 -> Visalization/Enable
  Saturation/1 -> Visalization/1(x), x/1, MATLAB Function/2(x)
  MATLAB Function/2(e) -> e/1

== system mci_models/Mechanical Systems/Lunar Lander ==
  q : Inport
  Integrator : Integrator  InitialCondition=x0
  MATLAB Function : MATLAB Function  TreatAsAtomicUnit=on
  Saturation : Saturate  UpperLimit=inf  LowerLimit=0
  x : Outport  VectorParamsAs1DForOutWhenUnconnected=off
  wires:
  MATLAB Function/1(xdot) -> Integrator/1
  Integrator/1 -> x/1, MATLAB Function/2(x)
  Saturation/1 -> MATLAB Function/1(u)
  q/1 -> Saturation/1

== system mci_models/Mechanical Systems/Segway Model ==
  M : Inport
  Integrator : Integrator  InitialCondition=x0
  MATLAB Function : MATLAB Function  TreatAsAtomicUnit=on
  display segway : Subsystem
  switch : Constant  Value=display
  x : Outport  VectorParamsAs1DForOutWhenUnconnected=off
  wires:
  switch/1 -> display segway/Enable
  MATLAB Function/1(dx) -> Integrator/1
  Integrator/1 -> MATLAB Function/2(x), x/1, display segway/1(x)
  M/1 -> MATLAB Function/1(u)

== system mci_models/Pendula/Double Pendulum on Cart ==
  F : Inport
  Enabled Subsystem : Subsystem  TreatAsAtomicUnit=on
  Integrator : Integrator  InitialCondition=x0
  MATLAB Function : MATLAB Function  TreatAsAtomicUnit=on
  switch : Constant  Value=display
  x : Outport  VectorParamsAs1DForOutWhenUnconnected=off
  wires:
  switch/1 -> Enabled Subsystem/Enable
  F/1 -> MATLAB Function/1(u), Enabled Subsystem/2(F)
  Integrator/1 -> MATLAB Function/2(x), x/1, Enabled Subsystem/1(x)
  MATLAB Function/1(xdot) -> Integrator/1

== system mci_models/Pendula/Mathematical Pendulum ==
  M : Inport
  Integrator : Integrator  InitialCondition=x0
  MATLAB Function : MATLAB Function  TreatAsAtomicUnit=on
  Visualization : Subsystem
  switch : Constant  Value=display
  x : Outport  VectorParamsAs1DForOutWhenUnconnected=off
  wires:
  MATLAB Function/1(xdot) -> Integrator/1
  M/1 -> MATLAB Function/1(u)
  Integrator/1 -> Visualization/1(x), MATLAB Function/2(x), x/1
  switch/1 -> Visualization/Enable

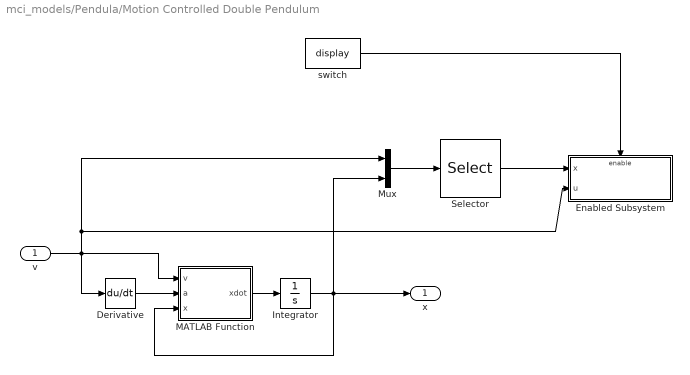
== system mci_models/Pendula/Motion Controlled Double Pendulum ==
  v : Inport
  Derivative : Derivative
  Enabled Subsystem : Subsystem  TreatAsAtomicUnit=on
  Integrator : Integrator  InitialCondition=x0
  MATLAB Function : MATLAB Function  TreatAsAtomicUnit=on
  Mux : Mux  Inputs=2
  Selector : Selector  InputPortWidth=6  IndexOptions=Index vector (dialog)  Indices=[2 3 4 1 5 6]  OutputSizes=1
  switch : Constant  Value=display
  x : Outport  VectorParamsAs1DForOutWhenUnconnected=off
  wires:
  switch/1 -> Enabled Subsystem/Enable
  v/1 -> Derivative/1, MATLAB Function/1(v), Mux/1, Enabled Subsystem/2(u)
  Integrator/1 -> Mux/2, MATLAB Function/3(x), x/1
  MATLAB Function/1(xdot) -> Integrator/1
  Derivative/1 -> MATLAB Function/2(a)
  Mux/1 -> Selector/1
  Selector/1 -> Enabled Subsystem/1(x)

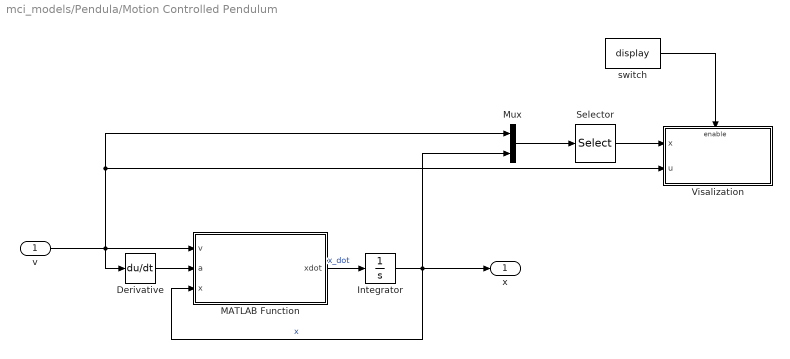
== system mci_models/Pendula/Motion Controlled Pendulum ==
  v : Inport
  Derivative : Derivative
  Integrator : Integrator  InitialCondition=x0
  MATLAB Function : MATLAB Function  TreatAsAtomicUnit=on
  Mux : Mux  Inputs=2
  Selector : Selector  InputPortWidth=4  IndexOptions=Index vector (dialog)  Indices=[2 3 1 4]  OutputSizes=1
  Visalization : Subsystem  TreatAsAtomicUnit=on
  switch : Constant  Value=display
  x : Outport  VectorParamsAs1DForOutWhenUnconnected=off
  wires:
  v/1 -> Visalization/2(u), Mux/1, Derivative/1, MATLAB Function/1(v)
  Integrator/1 -> Mux/2, x/1, MATLAB Function/3(x)  "x"
  MATLAB Function/1(xdot) -> Integrator/1  "x_dot"
  switch/1 -> Visalization/Enable
  Derivative/1 -> MATLAB Function/2(a)
  Mux/1 -> Selector/1
  Selector/1 -> Visalization/1(x)

== system mci_models/Pendula/Pendulum on Cart ==
  F : Inport
  Integrator : Integrator  InitialCondition=x0
  MATLAB Function : MATLAB Function  TreatAsAtomicUnit=on
  Visalization : Subsystem  TreatAsAtomicUnit=on
  switch : Constant  Value=display
  x : Outport  VectorParamsAs1DForOutWhenUnconnected=off
  wires:
  F/1 -> Visalization/2(u), MATLAB Function/1(F)
  Integrator/1 -> Visalization/1(x), x/1, MATLAB Function/2(x)  "x"
  MATLAB Function/1(xdot) -> Integrator/1  "x_dot"
  switch/1 -> Visalization/Enable

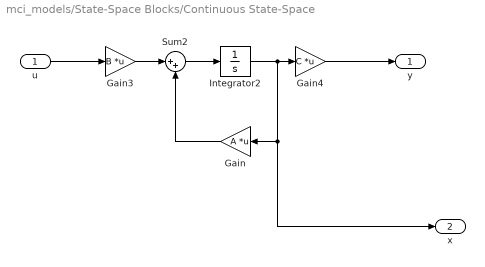
== system mci_models/State-Space Blocks/Continuous State-Space ==
  u : Inport
  Gain : Gain  Gain=A  Multiplication=Matrix(K*u)
  Gain3 : Gain  Gain=B  Multiplication=Matrix(K*u)
  Gain4 : Gain  Gain=C  Multiplication=Matrix(K*u)
  Integrator2 : Integrator  InitialCondition=x0
  Sum2 : Sum  Inputs=|++
  y : Outport  VectorParamsAs1DForOutWhenUnconnected=off
  x : Outport  Port=2  VectorParamsAs1DForOutWhenUnconnected=off
  wires:
  Integrator2/1 -> Gain4/1, Gain/1, x/1
  Gain3/1 -> Sum2/1
  Gain/1 -> Sum2/2
  Sum2/1 -> Integrator2/1
  Gain4/1 -> y/1
  u/1 -> Gain3/1

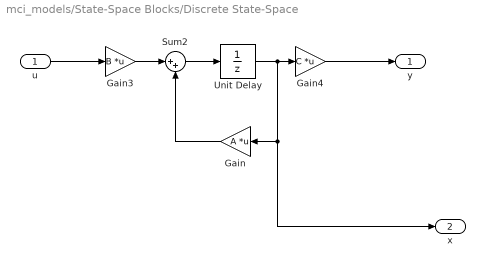
== system mci_models/State-Space Blocks/Discrete State-Space ==
  u : Inport
  Gain : Gain  Gain=A  Multiplication=Matrix(K*u)
  Gain3 : Gain  Gain=B  Multiplication=Matrix(K*u)
  Gain4 : Gain  Gain=C  Multiplication=Matrix(K*u)
  Sum2 : Sum  Inputs=|++
  Unit Delay : UnitDelay  InitialCondition=x0  SampleTime=T  HasFrameUpgradeWarning=on
  y : Outport  VectorParamsAs1DForOutWhenUnconnected=off
  x : Outport  Port=2  VectorParamsAs1DForOutWhenUnconnected=off
  wires:
  Unit Delay/1 -> Gain4/1, Gain/1, x/1
  Gain3/1 -> Sum2/1
  Gain/1 -> Sum2/2
  Sum2/1 -> Unit Delay/1
  Gain4/1 -> y/1
  u/1 -> Gain3/1

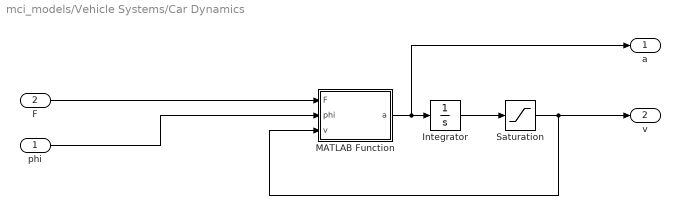
== system mci_models/Vehicle Systems/Car Dynamics ==
  phi : Inport
  F : Inport  Port=2
  Integrator : Integrator  InitialCondition=x0
  MATLAB Function : MATLAB Function  TreatAsAtomicUnit=on
  Saturation : Saturate  UpperLimit=inf  LowerLimit=0
  a : Outport  VectorParamsAs1DForOutWhenUnconnected=off
  v : Outport  Port=2  VectorParamsAs1DForOutWhenUnconnected=off
  wires:
  phi/1 -> MATLAB Function/2(phi)
  MATLAB Function/1(a) -> a/1, Integrator/1
  Integrator/1 -> Saturation/1
  F/1 -> MATLAB Function/1(F)
  Saturation/1 -> v/1, MATLAB Function/3(v)

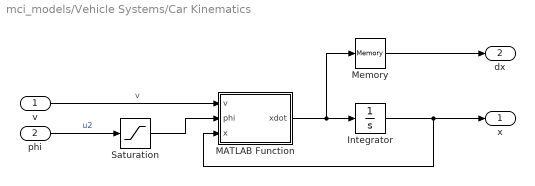
== system mci_models/Vehicle Systems/Car Kinematics ==
  v : Inport
  phi : Inport  Port=2
  Integrator : Integrator  InitialCondition=x0
  MATLAB Function : MATLAB Function  TreatAsAtomicUnit=on
  Memory : Memory
  Saturation : Saturate  UpperLimit=phimax  LowerLimit=-phimax
  x : Outport  VectorParamsAs1DForOutWhenUnconnected=off
  dx : Outport  Port=2  VectorParamsAs1DForOutWhenUnconnected=off
  wires:
  Integrator/1 -> MATLAB Function/3(x), x/1
  phi/1 -> Saturation/1  "u2"
  v/1 -> MATLAB Function/1(v)  "v"
  MATLAB Function/1(xdot) -> Memory/1, Integrator/1
  Memory/1 -> dx/1
  Saturation/1 -> MATLAB Function/2(phi)

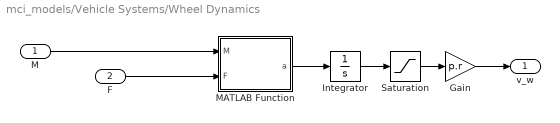
== system mci_models/Vehicle Systems/Wheel Dynamics ==
  M : Inport
  F : Inport  Port=2
  Gain : Gain  Gain=p.r
  Integrator : Integrator  InitialCondition=w0
  MATLAB Function : MATLAB Function  TreatAsAtomicUnit=on
  Saturation : Saturate  UpperLimit=inf  LowerLimit=0
  v_w : Outport  VectorParamsAs1DForOutWhenUnconnected=off
  wires:
  M/1 -> MATLAB Function/1(M)
  MATLAB Function/1(a) -> Integrator/1
  F/1 -> MATLAB Function/2(F)
  Gain/1 -> v_w/1
  Integrator/1 -> Saturation/1
  Saturation/1 -> Gain/1

== system mci_models/Fluid Systems/Fan Model/Sensor1 ==
  w : Inport
  Integrator : Integrator
  Pulse Generator : DiscretePulseGenerator  PulseType=Time based  Period=T  PulseWidth=5
  Quantizer : Quantizer  QuantizationInterval=pi/2
  Triggered Subsystem : Subsystem  TreatAsAtomicUnit=on
  w1 : Outport
  wires:
  Integrator/1 -> Quantizer/1
  Quantizer/1 -> Triggered Subsystem/1(u)
  Pulse Generator/1 -> Triggered Subsystem/Trigger
  Triggered Subsystem/1(w1) -> w1/1
  w/1 -> Integrator/1

== system mci_models/Fluid Systems/Fan Model/Sensor2 ==
  w : Inport
  Integrator : Integrator
  Pulse Generator : DiscretePulseGenerator  PulseType=Time based  Period=T  PulseWidth=5
  Quantizer : Quantizer  QuantizationInterval=pi/2
  Triggered Subsystem : Subsystem  TreatAsAtomicUnit=on
  w2 : Outport
  wires:
  Integrator/1 -> Quantizer/1
  Quantizer/1 -> Triggered Subsystem/1(u)
  Pulse Generator/1 -> Triggered Subsystem/Trigger
  Triggered Subsystem/1(w1) -> w2/1
  w/1 -> Integrator/1

== system mci_models/Mechanical Systems/Elevator/Visalization ==
  x : Inport
  Enable : EnablePort
  S-Function1 : S-Function  FunctionName=elevator_display  Parameters=display  SFunctionDeploymentMode=off  EnableBusSupport=off
  wires:
  x/1 -> S-Function1/1

== system mci_models/Mechanical Systems/Segway Model/display segway ==
  x : Inport
  Enable : EnablePort
  S-Function1 : S-Function  FunctionName=segway_display  Parameters=display  SFunctionDeploymentMode=off  EnableBusSupport=off
  wires:
  x/1 -> S-Function1/1

== system mci_models/Pendula/Double Pendulum on Cart/Enabled Subsystem ==
  x : Inport
  F : Inport  Port=2
  Enable : EnablePort
  Mux : Mux  Inputs=2
  S-Function : S-Function  FunctionName=double_pendulum_display  Parameters=display  SFunctionDeploymentMode=off  EnableBusSupport=off
  wires:
  F/1 -> Mux/2
  Mux/1 -> S-Function/1
  x/1 -> Mux/1

== system mci_models/Pendula/Mathematical Pendulum/Visualization ==
  x : Inport
  Enable : EnablePort
  S-Function : S-Function  FunctionName=pendulum_display  Parameters=display  SFunctionDeploymentMode=off  EnableBusSupport=off
  Selector : Selector  InputPortWidth=2  IndexOptions=Index vector (dialog)  Indices=[1]  OutputSizes=1
  wires:
  x/1 -> Selector/1
  Selector/1 -> S-Function/1

== system mci_models/Pendula/Motion Controlled Double Pendulum/Enabled Subsystem ==
  x : Inport
  u : Inport  Port=2
  Enable : EnablePort
  Mux : Mux  Inputs=2
  S-Function : S-Function  FunctionName=double_pendulum_display  Parameters=display  SFunctionDeploymentMode=off  EnableBusSupport=off
  wires:
  u/1 -> Mux/2
  Mux/1 -> S-Function/1
  x/1 -> Mux/1

== system mci_models/Pendula/Motion Controlled Pendulum/Visalization ==
  x : Inport
  u : Inport  Port=2
  Enable : EnablePort
  Mux : Mux  Inputs=2
  S-Function1 : S-Function  FunctionName=pendulum_cart_display  Parameters=display  SFunctionDeploymentMode=off  EnableBusSupport=off
  wires:
  u/1 -> Mux/2
  x/1 -> Mux/1
  Mux/1 -> S-Function1/1

== system mci_models/Pendula/Pendulum on Cart/Visalization ==
  x : Inport
  u : Inport  Port=2
  Enable : EnablePort
  Mux : Mux  Inputs=2
  S-Function1 : S-Function  FunctionName=pendulum_cart_display  Parameters=display  SFunctionDeploymentMode=off  EnableBusSupport=off
  wires:
  u/1 -> Mux/2
  x/1 -> Mux/1
  Mux/1 -> S-Function1/1

== system mci_models/Fluid Systems/Fan Model/Sensor1/Triggered Subsystem ==
  u : Inport
  Trigger : TriggerPort  VariantControl=(inherit)
  MATLAB Function : MATLAB Function  TreatAsAtomicUnit=on
  w1 : Outport
  wires:
  u/1 -> MATLAB Function/1(phi)
  MATLAB Function/1(w) -> w1/1

== system mci_models/Fluid Systems/Fan Model/Sensor2/Triggered Subsystem ==
  u : Inport
  Trigger : TriggerPort  VariantControl=(inherit)
  MATLAB Function : MATLAB Function  TreatAsAtomicUnit=on
  w1 : Outport
  wires:
  u/1 -> MATLAB Function/1(phi)
  MATLAB Function/1(w) -> w1/1

== matlab function mci_models/Fluid Systems/Bioreactor/MATLAB Function ==
  data: u input; xdot output; x input; p parameter
function xdot = fcn(u,x,p)

xdot=zeros(size(x));

mu=p.mu0*x(2)/(p.k0+p.k1*x(2)+p.k2*x(2)^2);

xdot(1)=(mu-u)*x(1);
xdot(2)=(p.cg0-x(2))*u-mu*x(1)/p.alpha;

== matlab function mci_models/Pendula/Double Pendulum on Cart/MATLAB Function ==
  data: u input; xdot output; x input; p parameter
function xdot = fcn(u,x,p)

dphi=x(3)-x(2);

FR=p.b0*x(4);
MR1=p.b1*x(5);
MR2=p.b2*(x(6)-x(5));

a=p.M;
b=p.I12p*cos(x(2));
c=p.I2p*cos(x(3));
e=p.I11;
f=p.I12*cos(dphi);
i=p.I22;

mi11=e*i-f^2;
mi12=c*f-b*i;
mi13=b*f-c*e;
mi22=a*i-c^2;
mi23=b*c-a*f;
mi33=a*e-b^2;

Mi=[mi11 mi12 mi13;mi12 mi22 mi23;mi13 mi23 mi33];
D=[-p.I12p*sin(x(2)) -p.I2p*sin(x(3)) 0; ...
    0 -p.I12*sin(dphi) p.I12p*sin(x(2)); ...
    p.I12*sin(dphi) 0 p.I2p*sin(x(3))];

q=Mi*([u-FR;MR2-MR1;-MR2]-D*[x(5)^2;x(6)^2;p.g])/(mi33*i+mi23*f+mi13*c);

xdot=[x(4:6);q];

== matlab function mci_models/Pendula/Motion Controlled Double Pendulum/MATLAB Function ==
  data: v input; a input; xdot output; x input; p parameter
function xdot = fcn(v,a,x,p)

xdot=zeros(size(x));

dphi=x(3)-x(2);

MR1=p.b1*x(4);
MR2=p.b2*(x(5)-x(4));

Mi=[p.I22 -p.I12*cos(dphi);-p.I12*cos(dphi) p.I11]/(p.I11*p.I22-(p.I12*cos(dphi))^2);
D1=[0 -p.I12*sin(dphi);p.I12*sin(dphi) 0];
D2=[p.I12p*cos(x(2)) p.I12p*sin(x(2));p.I2p*cos(x(3)) p.I2p*sin(x(3))];

q=Mi*([MR2-MR1;-MR2]-D1*[x(4)^2;x(5)^2]-D2*[a;p.g]);

xdot=[v;x(4:5);q];

== matlab function mci_models/Electric Systems/Magnetic Levitation/MATLAB Function ==
  data: u input; xdot output size=[3,1]; x input; p parameter
function xdot = fcn(u,x,p)

xdot=zeros(size(x));

xdot(1)=x(2);
xdot(2)=p.g-p.L1*x(3)^2/(2*p.m*p.y0*(1+x(1)/p.y0)^2);
xdot(3)=(u-(p.R-p.L1*x(2)/((1+x(1)/p.y0)^2*p.y0))*x(3))/(p.L0+p.L1/(1+x(1)/p.y0));
%xdot(3)=(u-p.R*x(3))/(p.L0+p.L1/(1+x(1)/p.y0));

== matlab function mci_models/Fluid Systems/Pneumatic Cylinder/MATLAB Function ==
  data: u input; dx output; x input; p parameter
function dx = fcn(u,x,p)
%#codegen

dx=zeros(size(x));

dx(1) = x(2);
dx(2) = (p.A*x(3)-p.b*x(2)-p.k*x(1))/p.m;
dx(3) = x(3)/x(1)*(u/p.A-x(2));

== matlab function mci_models/Mechanical Systems/Elevator/MATLAB Function ==
  data: M input; xdot output; x input; p parameter; e output
function [xdot,e] = pendulum_model(M,x,p)

% x=[y;phi;ydot;phidot]

xdot=zeros(size(x));

Fr=p.b1*x(3);
Mr=p.b2*x(4);
l=p.r*x(2);
e=max(0,(x(1)-l)/(l));
Fs=e*p.k;

xdot(1)=x(3);
xdot(2)=x(4);
xdot(3)=p.g-(Fs+Fr)/p.m;
xdot(4)=(Fs*p.r+M-Mr)/p.J;
